simulink model "daolibai1"  (R2023b)
settings: Solver=FixedStepAuto  StartTime=0.0  StopTime=10.0  FixedStep=0.01  RelTol=1e-3
settings Model: Creator=asus  LastModifiedBy=asus

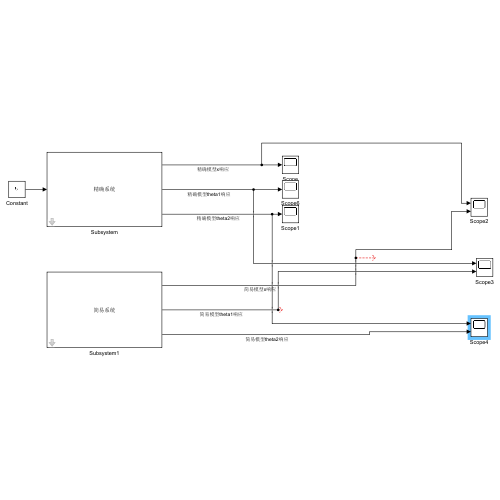
[thumbnail: Simulink's stored preview of the top-level diagram]
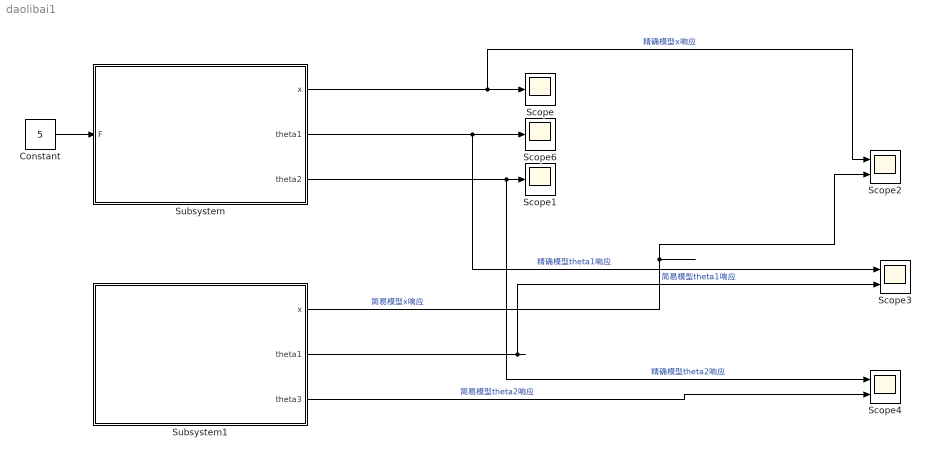
== system daolibai1 ==
  Constant : Constant  Value=5
  Scope : Scope
  Scope1 : Scope
  Scope2 : Scope  NumInputPorts=2
  Scope3 : Scope  NumInputPorts=2
  Scope4 : Scope  NumInputPorts=2
  Scope6 : Scope
  Subsystem : Subsystem  mask{M=1, m1=0.5, m2=0.5, L1=0.6, L2=0.6, g=9.8, theta10=0, theta20=0, x0=0}
      mask prompts: theta10 "theta1(0)"; theta20 "tehta2(0)"
      mask DialogControl ParameterGroupVar Prompt: 参数
      mask Display: disp('精确系统');
  Subsystem1 : Subsystem  mask{M=1, m1=0.5, m2=0.5, L1=0.6, L2=0.6, g=9.8, theta10=0, theta20=0, x0=0, F=5}
      mask prompts: theta10 "theta1(0)"; theta20 "tehta2(0)"
      mask DialogControl ParameterGroupVar Prompt: 参数
      mask Display: disp('简易系统');
  wires:
  Constant/1 -> Subsystem/1(F)
  Subsystem/1(x) -> Scope2/1, Scope/1  "精确模型x响应"
  Subsystem/2(theta1) -> Scope3/1, Scope6/1  "精确模型theta1响应"
  Subsystem/3(theta2) -> Scope4/1, Scope1/1  "精确模型theta2响应"
  Subsystem1/3(theta3) -> Scope4/2  "简易模型theta2响应"
  Subsystem1/2(theta1) -> Scope3/2  "简易模型theta1响应"
  Subsystem1/1(x) -> Scope2/2  "简易模型x响应"

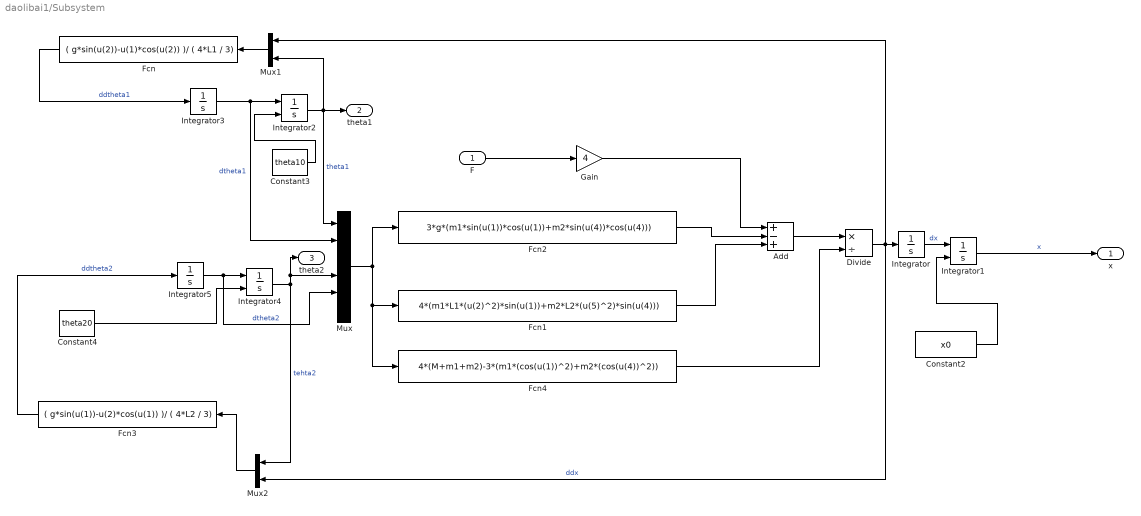
== system daolibai1/Subsystem ==
  F : Inport
  Add : Sum  Inputs=+-+
  Constant2 : Constant  Value=x0
  Constant3 : Constant  Value=theta10
  Constant4 : Constant  Value=theta20
  Divide : Product  Inputs=*/
  Fcn : Fcn  Expr=( g*sin(u(2))-u(1)*cos(u(2)) )/ ( 4*L1 / 3)
  Fcn1 : Fcn  Expr=4*(m1*L1*(u(2)^2)*sin(u(1))+m2*L2*(u(5)^2)*sin(u(4)))
  Fcn2 : Fcn  Expr=3*g*(m1*sin(u(1))*cos(u(1))+m2*sin(u(4))*cos(u(4)))
  Fcn3 : Fcn  Expr=( g*sin(u(1))-u(2)*cos(u(1)) )/ ( 4*L2 / 3)
  Fcn4 : Fcn  Expr=4*(M+m1+m2)-3*(m1*(cos(u(1))^2)+m2*(cos(u(4))^2))
  Gain : Gain  Gain=4
  Integrator : Integrator
  Integrator1 : Integrator  InitialConditionSource=external
  Integrator2 : Integrator  InitialConditionSource=external
  Integrator3 : Integrator
  Integrator4 : Integrator  InitialConditionSource=external
  Integrator5 : Integrator
  Mux : Mux  Inputs=6
  Mux1 : Mux  Inputs=2
  Mux2 : Mux  Inputs=2
  x : Outport
  theta1 : Outport  Port=2
  theta2 : Outport  Port=3
  wires:
  Integrator/1 -> Integrator1/1  "dx"
  Integrator3/1 -> Mux/2, Integrator2/1  "dtheta1"
  Fcn3/1 -> Integrator5/1  "ddtheta2"
  Mux2/1 -> Fcn3/1
  Mux/1 -> Fcn4/1, Fcn1/1, Fcn2/1
  Integrator5/1 -> Mux/5, Integrator4/1  "dtheta2"
  Fcn2/1 -> Add/2
  Fcn/1 -> Integrator3/1  "ddtheta1"
  Divide/1 -> Mux2/2, Integrator/1, Mux1/1  "ddx"
  Integrator2/1 -> theta1/1, Mux1/2, Mux/1  "theta1"
  Integrator4/1 -> theta2/1, Mux/4, Mux2/1  "tehta2"
  F/1 -> Gain/1
  Mux1/1 -> Fcn/1
  Fcn1/1 -> Add/3
  Integrator1/1 -> x/1  "x"
  Constant2/1 -> Integrator1/2
  Add/1 -> Divide/1
  Constant3/1 -> Integrator2/2
  Constant4/1 -> Integrator4/2
  Gain/1 -> Add/1
  Fcn4/1 -> Divide/2

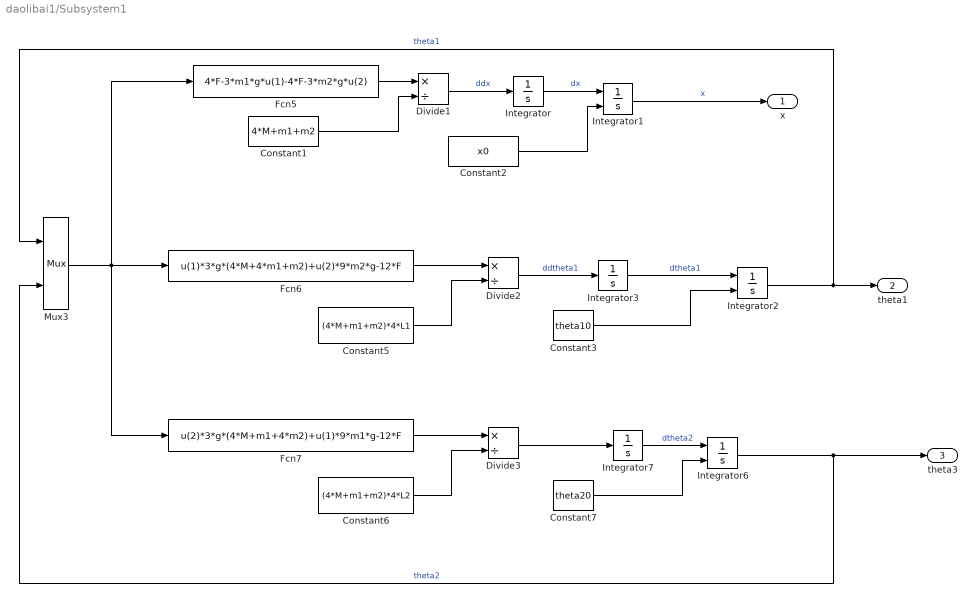
== system daolibai1/Subsystem1 ==
  Constant1 : Constant  Value=4*M+m1+m2
  Constant2 : Constant  Value=x0
  Constant3 : Constant  Value=theta10
  Constant5 : Constant  Value=(4*M+m1+m2)*4*L1
  Constant6 : Constant  Value=(4*M+m1+m2)*4*L2
  Constant7 : Constant  Value=theta20
  Divide1 : Product  Inputs=*/
  Divide2 : Product  Inputs=*/
  Divide3 : Product  Inputs=*/
  Fcn5 : Fcn  Expr=4*F-3*m1*g*u(1)-4*F-3*m2*g*u(2)
  Fcn6 : Fcn  Expr=u(1)*3*g*(4*M+4*m1+m2)+u(2)*9*m2*g-12*F
  Fcn7 : Fcn  Expr=u(2)*3*g*(4*M+m1+4*m2)+u(1)*9*m1*g-12*F
  Integrator : Integrator
  Integrator1 : Integrator  InitialConditionSource=external
  Integrator2 : Integrator  InitialConditionSource=external
  Integrator3 : Integrator
  Integrator6 : Integrator  InitialConditionSource=external
  Integrator7 : Integrator
  Mux3 : Mux  Inputs=2
  x : Outport
  theta1 : Outport  Port=2
  theta3 : Outport  Port=3
  wires:
  Integrator2/1 -> Mux3/1, theta1/1  "theta1"
  Integrator6/1 -> Mux3/2, theta3/1  "theta2"
  Fcn5/1 -> Divide1/1
  Constant1/1 -> Divide1/2
  Divide1/1 -> Integrator/1  "ddx"
  Constant2/1 -> Integrator1/2
  Integrator1/1 -> x/1  "x"
  Integrator/1 -> Integrator1/1  "dx"
  Fcn6/1 -> Divide2/1
  Constant5/1 -> Divide2/2
  Constant3/1 -> Integrator2/2
  Divide2/1 -> Integrator3/1  "ddtheta1"
  Integrator3/1 -> Integrator2/1  "dtheta1"
  Fcn7/1 -> Divide3/1
  Mux3/1 -> Fcn7/1, Fcn6/1, Fcn5/1
  Constant6/1 -> Divide3/2
  Integrator7/1 -> Integrator6/1  "dtheta2"
  Divide3/1 -> Integrator7/1
  Constant7/1 -> Integrator6/2
